simulink model "SD_NL_TORA"  (R2019b)
settings: Solver=ode4  StartTime=0.0  StopTime=stoptime  FixedStep=h  RelTol=1e-6  AbsTol=1e-6  EnableMultiTasking=on
values from neighbouring files (symbols this model uses):
  A = [0, 1, 0, 0 ... (first row only)    [mainfile_solution.m]
  B = [0 ... (first row only)    [mainfile_solution.m]
  C = eye(4)    [mainfile_solution.m]
  D = zeros(4,1)    [mainfile_solution.m]
  Kd = place(Ad,Bd,p_z)    [mainfile_solution.m]
  x0 = [20*pi/180 , 0 ,  0.1 , 0]'    [mainfile_solution.m]
  x0_tilde = x0 - x_bar    [mainfile_solution.m]
  x_bar = [0 0 0 0]'    [mainfile_solution.m]
settings Model: Creator=Ale  LastModifiedBy=don
settings SolverCC: AutoScaleAbsTol=off
settings DataIOCC: SaveFormat=Array  SignalLoggingSaveFormat=ModelDataLogs  SaveOutput=off  SaveTime=off  TimeSaveName=t
settings OptimizationCC: ExpressionDepthLimit=2147483647  LifeSpan=inf
settings DebuggingCC: UnderspecifiedInitializationDetection=Classic  MergeDetectMultiDrivingBlocksExec=none  FcnCallInpInsideContextMsg=warning  StateNameClashWarn=warning  SFUnexpectedBacktrackingDiag=warning  SFNoUnconditionalDefaultTransitionDiag=warning  SFExecutionAtInitializationDiag=none  ArithmeticOperatorsInVariantConditions=warning
settings HardwareCC: ProdBitPerPointer=32  ProdBitPerSizeT=32  ProdBitPerPtrDiffT=32  ProdLargestAtomicFloat=None  ProdIntDivRoundTo=Undefined  ProdEndianess=Unspecified  ProdWordSize=32  ProdHWDeviceType=32-bit Generic
settings ModelReferenceCC: PropagateSignalLabelsOutOfModel=off
settings SFSimCC: SimUseLocalCustomCode=off  CustomCodeUndefinedFunction=UseInterfaceOnly
settings RTWCC: RTWUseLocalCustomCode=off
settings CodeAppCC: StateflowObjectComments=on
settings GRTTargetCC: TargetLangStandard=C89/C90 (ANSI)  GeneratePreprocessorConditionals=Disable all  CombineOutputUpdateFcns=off  GRTInterface=on
settings ConfigComp: CovMetricSettings=dw  CovHtmlReporting=on  CovSaveCumulativeToWorkspaceVar=on  CovSaveSingleToWorkspaceVar=on  CovExternalEMLEnable=off

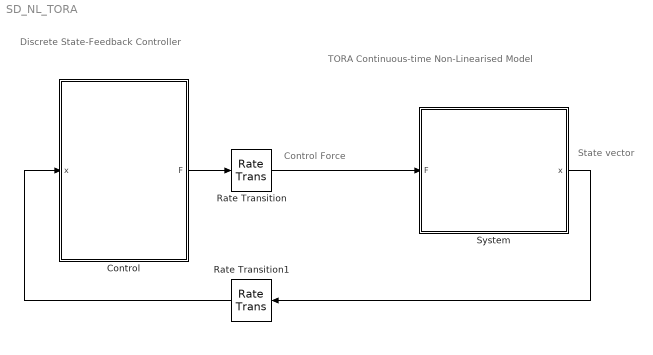
== system SD_NL_TORA ==
  note: Discrete State-Feedback
      | Controller
  note: Control Force
  note: State vector
  note: TORA
      | Continuous-time Non-Linearised Model
  Control : Subsystem
  Rate Transition : RateTransition  InitialCondition=-Kd*x0_tilde
  Rate Transition1 : RateTransition  InitialCondition=x0_tilde  OutPortSampleTime=Ts
  System : Subsystem
  wires:
  Control/1(F) -> Rate Transition/1
  Rate Transition/1 -> System/1(F)
  System/1(x) -> Rate Transition1/1
  Rate Transition1/1 -> Control/1(x)

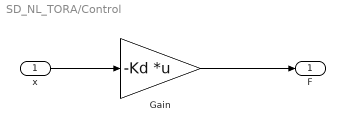
== system SD_NL_TORA/Control ==
  x : Inport
  Gain : Gain  Gain=-Kd  Multiplication=Matrix(K*u)
  F : Outport  VectorParamsAs1DForOutWhenUnconnected=off
  wires:
  x/1 -> Gain/1
  Gain/1 -> F/1

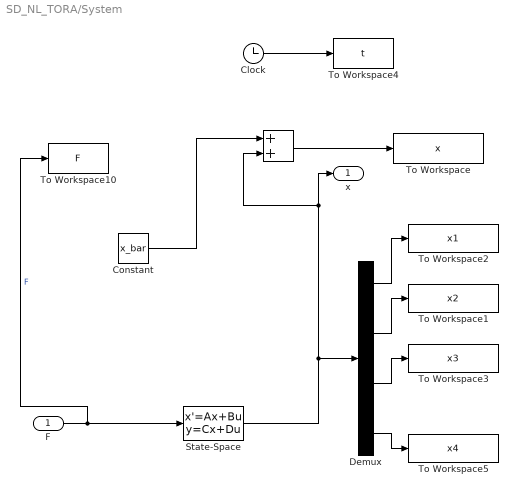
== system SD_NL_TORA/System ==
  F : Inport
  " " : Sum
  Clock : Clock
  Constant : Constant  Value=x_bar
  Demux : Demux
  State-Space : StateSpace  A=A  B=B  C=C  D=D  InitialCondition=x0
  To Workspace : ToWorkspace  VariableName=x  SampleTime=-1
  To Workspace1 : ToWorkspace  VariableName=x2  SampleTime=-1
  To Workspace10 : ToWorkspace  VariableName=F  SampleTime=-1
  To Workspace2 : ToWorkspace  VariableName=x1  SampleTime=-1
  To Workspace3 : ToWorkspace  VariableName=x3  SampleTime=-1
  To Workspace4 : ToWorkspace  VariableName=t  SampleTime=-1
  To Workspace5 : ToWorkspace  VariableName=x4  SampleTime=-1
  x : Outport  VectorParamsAs1DForOutWhenUnconnected=off
  wires:
  State-Space/1 -> x/1, " "/2, Demux/1
  Clock/1 -> To Workspace4/1
  F/1 -> State-Space/1, To Workspace10/1  "F"
  Constant/1 -> " "/1
  " "/1 -> To Workspace/1
  Demux/3 -> To Workspace3/1
  Demux/2 -> To Workspace1/1
  Demux/1 -> To Workspace2/1
  Demux/4 -> To Workspace5/1
